simulink model "PID_Controller"  (R2020b)
settings: Solver=VariableStepAuto  StartTime=0.0  StopTime=10.0  RelTol=1e-3
undefined symbols (not defined in the file or in its folder): Kd, Ki, Kp
settings Model: Creator=shoun  LastModifiedBy=shoun

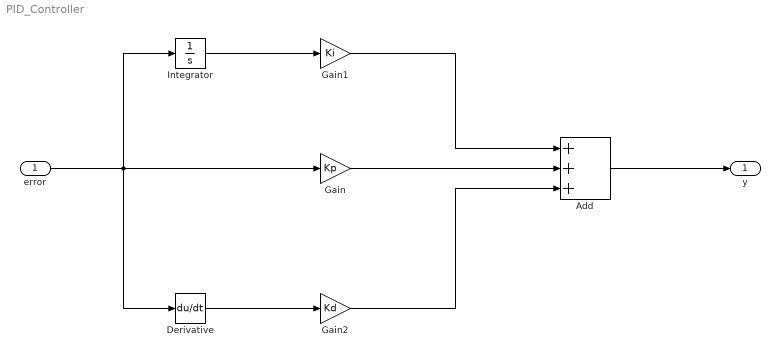
== system PID_Controller ==
  error : Inport  OutDataTypeStr=double  PortDimensions=1  SampleTime=0
  Add : Sum  Inputs=+++
  Derivative : Derivative
  Gain : Gain  Gain=Kp
  Gain1 : Gain  Gain=Ki
  Gain2 : Gain  Gain=Kd
  Integrator : Integrator
  y : Outport  OutDataTypeStr=double  PortDimensions=1  SampleTime=0
  wires:
  Gain1/1 -> Add/1
  Gain/1 -> Add/2
  Gain2/1 -> Add/3
  error/1 -> Gain/1, Integrator/1, Derivative/1
  Derivative/1 -> Gain2/1
  Add/1 -> y/1
  Integrator/1 -> Gain1/1
